simulink model "generic_IsaacV3"  (R2015a)
settings: Solver=ode3  StartTime=0.0  StopTime=inf  FixedStep=0.001  RelTol=1e-3
values from neighbouring files (symbols this model uses):
  coast_domain = 0.1    [LoadVar.m]
  DifferentialFactor = 0.5    [LoadVar.m]
  g = 9.81    [LoadVar.m]
  GearRatio = 10.364    [LoadVar.m]
  Gr = 10.32    [LoadVar.m]
  Lf = 0.78    [LoadVar.m]
  Lr = 0.745    [LoadVar.m]
  M = 265    [LoadVar.m]
  max_coast_Nm = 0    [LoadVar.m]
  MaxSteeringAngle = 24.635    [LoadVar.m]
  mu_max = 1.5    [LoadVar.m]
  ped_max_limiet = 1    [LoadVar.m]
  pedal_position_maxacc = 0.9    [LoadVar.m]
  Reff = 0.2325    [LoadVar.m]
  regen_activation_kph = 15    [LoadVar.m]
  slewbreak_domain = 0.15    [LoadVar.m]
  Sr = 0.6    [LoadVar.m]
  T_max_Nm = 40    [LoadVar.m]
  T_min_Nm = -15    [LoadVar.m]
  TireRadius = 0.4572/2    (= 0.2286)    [LoadVar.m]
  Tmax = 40    [LoadVar.m]
  TrackLength = 1.534    [LoadVar.m]
  TrackWidth = 1.200    (= 1.2)    [LoadVar.m]
libraries: CarMaker4SL x21, simulink x7
(part 3 of 3)

== system generic_IsaacV3/CarMaker/IPG Vehicle/CarAndTrailer/Trailer/CreateBus Vhcl.Wheel.FR ==
  In1 : Inport
  Bus Creator3 : BusCreator  Inputs=14
  Demux3 : Demux  Outputs=14
  Out1 : Outport
  wires:
  Demux3/14 -> Bus Creator3/14  "Vhcl Wheel FR Trq_WhlBearing"
  Demux3/13 -> Bus Creator3/13  "Vhcl Wheel FR Trq_T2W"
  Demux3/12 -> Bus Creator3/12  "Vhcl Wheel FR SideSlip"
  Demux3/11 -> Bus Creator3/11  "Vhcl Wheel FR LongSlip"
  Demux3/10 -> Bus Creator3/10  "Vhcl Wheel FR vBelt"
  Demux3/9 -> Bus Creator3/9  "Vhcl Wheel FR Fz"
  Demux3/8 -> Bus Creator3/8  "Vhcl Wheel FR Fy"
  Demux3/7 -> Bus Creator3/7  "Vhcl Wheel FR Fx"
  Demux3/6 -> Bus Creator3/6  "Vhcl Wheel FR r_zxy z"
  Demux3/5 -> Bus Creator3/5  "Vhcl Wheel FR r_zxy y"
  Demux3/4 -> Bus Creator3/4  "Vhcl Wheel FR r_zxy x"
  Demux3/3 -> Bus Creator3/3  "Vhcl Wheel FR t z"
  Demux3/2 -> Bus Creator3/2  "Vhcl Wheel FR t y"
  In1/1 -> Demux3/1
  Bus Creator3/1 -> Out1/1
  Demux3/1 -> Bus Creator3/1  "Vhcl Wheel FR t x"

== system generic_IsaacV3/CarMaker/IPG Vehicle/CarAndTrailer/Trailer/CreateBus Vhcl.Wheel.RL ==
  In1 : Inport
  Bus Creator3 : BusCreator  Inputs=14
  Demux3 : Demux  Outputs=14
  Out1 : Outport
  wires:
  Demux3/14 -> Bus Creator3/14  "Vhcl Wheel RL Trq_WhlBearing"
  Demux3/13 -> Bus Creator3/13  "Vhcl Wheel RL Trq_T2W"
  Demux3/12 -> Bus Creator3/12  "Vhcl Wheel RL SideSlip"
  Demux3/11 -> Bus Creator3/11  "Vhcl Wheel RL LongSlip"
  Demux3/10 -> Bus Creator3/10  "Vhcl Wheel RL vBelt"
  Demux3/9 -> Bus Creator3/9  "Vhcl Wheel RL Fz"
  Demux3/8 -> Bus Creator3/8  "Vhcl Wheel RL Fy"
  Demux3/7 -> Bus Creator3/7  "Vhcl Wheel RL Fx"
  Demux3/6 -> Bus Creator3/6  "Vhcl Wheel RL r_zxy z"
  Demux3/5 -> Bus Creator3/5  "Vhcl Wheel RL r_zxy y"
  Demux3/4 -> Bus Creator3/4  "Vhcl Wheel RL r_zxy x"
  Demux3/3 -> Bus Creator3/3  "Vhcl Wheel RL t z"
  Demux3/2 -> Bus Creator3/2  "Vhcl Wheel RL t y"
  In1/1 -> Demux3/1
  Bus Creator3/1 -> Out1/1
  Demux3/1 -> Bus Creator3/1  "Vhcl Wheel RL t x"

== system generic_IsaacV3/CarMaker/IPG Vehicle/CarAndTrailer/Trailer/CreateBus Vhcl.Wheel.RR ==
  In1 : Inport
  Bus Creator3 : BusCreator  Inputs=14
  Demux3 : Demux  Outputs=14
  Out1 : Outport
  wires:
  Demux3/14 -> Bus Creator3/14  "Vhcl Wheel RR Trq_WhlBearing"
  Demux3/13 -> Bus Creator3/13  "Vhcl Wheel RR Trq_T2W"
  Demux3/12 -> Bus Creator3/12  "Vhcl Wheel RR SideSlip"
  Demux3/11 -> Bus Creator3/11  "Vhcl Wheel RR LongSlip"
  Demux3/10 -> Bus Creator3/10  "Vhcl Wheel RR vBelt"
  Demux3/9 -> Bus Creator3/9  "Vhcl Wheel RR Fz"
  Demux3/8 -> Bus Creator3/8  "Vhcl Wheel RR Fy"
  Demux3/7 -> Bus Creator3/7  "Vhcl Wheel RR Fx"
  Demux3/6 -> Bus Creator3/6  "Vhcl Wheel RR r_zxy z"
  Demux3/5 -> Bus Creator3/5  "Vhcl Wheel RR r_zxy y"
  Demux3/4 -> Bus Creator3/4  "Vhcl Wheel RR r_zxy x"
  Demux3/3 -> Bus Creator3/3  "Vhcl Wheel RR t z"
  Demux3/2 -> Bus Creator3/2  "Vhcl Wheel RR t y"
  In1/1 -> Demux3/1
  Bus Creator3/1 -> Out1/1
  Demux3/1 -> Bus Creator3/1  "Vhcl Wheel RR t x"

== system generic_IsaacV3/CarMaker/TorqueVectoring/Post-processor/Fysische beperkingen/Lineaire programmering code ==
  Ground{,1..3} (4 alike) : Ground
  Lineaire programering : MATLAB Function  TreatAsAtomicUnit=on
  Terminator : Terminator
  Terminator1 : Terminator
  wires:
  Lineaire programering/2(Trr) -> Terminator1/1
  Lineaire programering/1(Trl) -> Terminator/1
  Ground/1 -> Lineaire programering/1(Trl_maxB)
  Ground2/1 -> Lineaire programering/3(Mz)
  Ground3/1 -> Lineaire programering/4(Tgevraagd)
  Ground1/1 -> Lineaire programering/2(Trr_maxB)

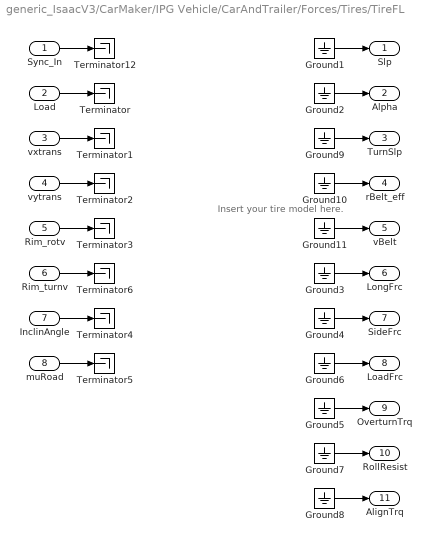
== system generic_IsaacV3/CarMaker/IPG Vehicle/CarAndTrailer/Forces/Tires/TireFL ==
  note: Insert your tire model here.
  Sync_In : Inport
  Load : Inport  Port=2
  vxtrans : Inport  Port=3
  vytrans : Inport  Port=4
  Rim_rotv : Inport  Port=5
  Rim_turnv : Inport  Port=6
  InclinAngle : Inport  Port=7
  muRoad : Inport  Port=8
  Ground{1..11} (11 alike) : Ground
  Terminator{,1..6,12} (8 alike) : Terminator
  Slp : Outport
  Alpha : Outport  Port=2
  TurnSlp : Outport  Port=3
  rBelt_eff : Outport  Port=4
  vBelt : Outport  Port=5
  LongFrc : Outport  Port=6
  SideFrc : Outport  Port=7
  LoadFrc : Outport  Port=8
  OverturnTrq : Outport  Port=9
  RollResist : Outport  Port=10
  AlignTrq : Outport  Port=11
  wires:
  Ground11/1 -> vBelt/1
  Ground10/1 -> rBelt_eff/1
  Ground9/1 -> TurnSlp/1
  Rim_turnv/1 -> Terminator6/1
  Sync_In/1 -> Terminator12/1
  Ground2/1 -> Alpha/1
  Ground3/1 -> LongFrc/1
  Ground4/1 -> SideFrc/1
  Ground5/1 -> OverturnTrq/1
  vxtrans/1 -> Terminator1/1
  vytrans/1 -> Terminator2/1
  Rim_rotv/1 -> Terminator3/1
  InclinAngle/1 -> Terminator4/1
  muRoad/1 -> Terminator5/1
  Load/1 -> Terminator/1
  Ground1/1 -> Slp/1
  Ground6/1 -> LoadFrc/1
  Ground7/1 -> RollResist/1
  Ground8/1 -> AlignTrq/1

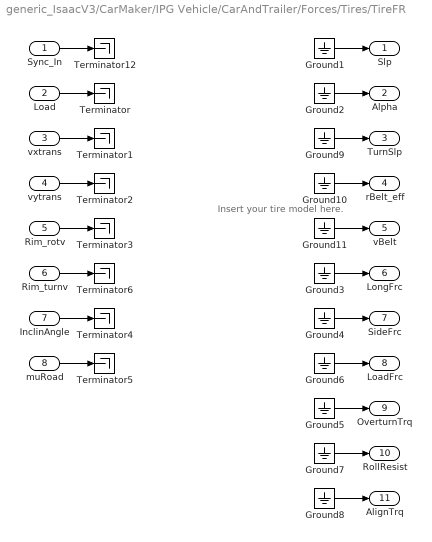
== system generic_IsaacV3/CarMaker/IPG Vehicle/CarAndTrailer/Forces/Tires/TireFR ==
  note: Insert your tire model here.
  Sync_In : Inport
  Load : Inport  Port=2
  vxtrans : Inport  Port=3
  vytrans : Inport  Port=4
  Rim_rotv : Inport  Port=5
  Rim_turnv : Inport  Port=6
  InclinAngle : Inport  Port=7
  muRoad : Inport  Port=8
  Ground{1..11} (11 alike) : Ground
  Terminator{,1..6,12} (8 alike) : Terminator
  Slp : Outport
  Alpha : Outport  Port=2
  TurnSlp : Outport  Port=3
  rBelt_eff : Outport  Port=4
  vBelt : Outport  Port=5
  LongFrc : Outport  Port=6
  SideFrc : Outport  Port=7
  LoadFrc : Outport  Port=8
  OverturnTrq : Outport  Port=9
  RollResist : Outport  Port=10
  AlignTrq : Outport  Port=11
  wires:
  Ground11/1 -> vBelt/1
  Ground10/1 -> rBelt_eff/1
  Ground9/1 -> TurnSlp/1
  Rim_turnv/1 -> Terminator6/1
  Sync_In/1 -> Terminator12/1
  Ground2/1 -> Alpha/1
  Ground3/1 -> LongFrc/1
  Ground4/1 -> SideFrc/1
  Ground5/1 -> OverturnTrq/1
  vxtrans/1 -> Terminator1/1
  vytrans/1 -> Terminator2/1
  Rim_rotv/1 -> Terminator3/1
  InclinAngle/1 -> Terminator4/1
  muRoad/1 -> Terminator5/1
  Load/1 -> Terminator/1
  Ground1/1 -> Slp/1
  Ground6/1 -> LoadFrc/1
  Ground7/1 -> RollResist/1
  Ground8/1 -> AlignTrq/1

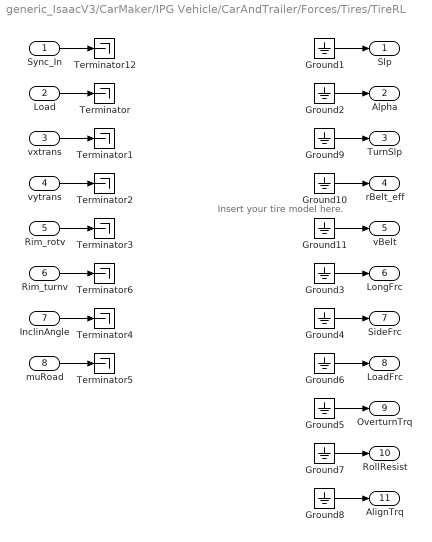
== system generic_IsaacV3/CarMaker/IPG Vehicle/CarAndTrailer/Forces/Tires/TireRL ==
  note: Insert your tire model here.
  Sync_In : Inport
  Load : Inport  Port=2
  vxtrans : Inport  Port=3
  vytrans : Inport  Port=4
  Rim_rotv : Inport  Port=5
  Rim_turnv : Inport  Port=6
  InclinAngle : Inport  Port=7
  muRoad : Inport  Port=8
  Ground{1..11} (11 alike) : Ground
  Terminator{,1..6,12} (8 alike) : Terminator
  Slp : Outport
  Alpha : Outport  Port=2
  TurnSlp : Outport  Port=3
  rBelt_eff : Outport  Port=4
  vBelt : Outport  Port=5
  LongFrc : Outport  Port=6
  SideFrc : Outport  Port=7
  LoadFrc : Outport  Port=8
  OverturnTrq : Outport  Port=9
  RollResist : Outport  Port=10
  AlignTrq : Outport  Port=11
  wires:
  Ground11/1 -> vBelt/1
  Ground10/1 -> rBelt_eff/1
  Ground9/1 -> TurnSlp/1
  Rim_turnv/1 -> Terminator6/1
  Sync_In/1 -> Terminator12/1
  Ground2/1 -> Alpha/1
  Ground3/1 -> LongFrc/1
  Ground4/1 -> SideFrc/1
  Ground5/1 -> OverturnTrq/1
  vxtrans/1 -> Terminator1/1
  vytrans/1 -> Terminator2/1
  Rim_rotv/1 -> Terminator3/1
  InclinAngle/1 -> Terminator4/1
  muRoad/1 -> Terminator5/1
  Load/1 -> Terminator/1
  Ground1/1 -> Slp/1
  Ground6/1 -> LoadFrc/1
  Ground7/1 -> RollResist/1
  Ground8/1 -> AlignTrq/1

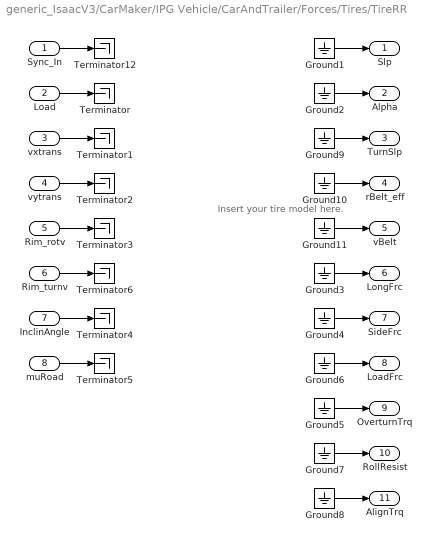
== system generic_IsaacV3/CarMaker/IPG Vehicle/CarAndTrailer/Forces/Tires/TireRR ==
  note: Insert your tire model here.
  Sync_In : Inport
  Load : Inport  Port=2
  vxtrans : Inport  Port=3
  vytrans : Inport  Port=4
  Rim_rotv : Inport  Port=5
  Rim_turnv : Inport  Port=6
  InclinAngle : Inport  Port=7
  muRoad : Inport  Port=8
  Ground{1..11} (11 alike) : Ground
  Terminator{,1..6,12} (8 alike) : Terminator
  Slp : Outport
  Alpha : Outport  Port=2
  TurnSlp : Outport  Port=3
  rBelt_eff : Outport  Port=4
  vBelt : Outport  Port=5
  LongFrc : Outport  Port=6
  SideFrc : Outport  Port=7
  LoadFrc : Outport  Port=8
  OverturnTrq : Outport  Port=9
  RollResist : Outport  Port=10
  AlignTrq : Outport  Port=11
  wires:
  Ground11/1 -> vBelt/1
  Ground10/1 -> rBelt_eff/1
  Ground9/1 -> TurnSlp/1
  Rim_turnv/1 -> Terminator6/1
  Sync_In/1 -> Terminator12/1
  Ground2/1 -> Alpha/1
  Ground3/1 -> LongFrc/1
  Ground4/1 -> SideFrc/1
  Ground5/1 -> OverturnTrq/1
  vxtrans/1 -> Terminator1/1
  vytrans/1 -> Terminator2/1
  Rim_rotv/1 -> Terminator3/1
  InclinAngle/1 -> Terminator4/1
  muRoad/1 -> Terminator5/1
  Load/1 -> Terminator/1
  Ground1/1 -> Slp/1
  Ground6/1 -> LoadFrc/1
  Ground7/1 -> RollResist/1
  Ground8/1 -> AlignTrq/1

== stateflow chart generic_IsaacV3/CarMaker/PedalMapping/Chart ==
  state LaunchSet
    entry:
    pedal=0;
    during:
    pedal=0;
    DRS_S2=0;
    DRS_S3=0;
  state LaunchGo
    during:
    pedal=ped_pos;
    DRS_S2=0;
    DRS_S3=0;
  (default) -> LaunchSet
  LaunchSet -> LaunchGo : [LC==1 && ped_pos>=0.8]
  LaunchGo -> LaunchSet : [LC==0]
  data: ped_pos input; pedal output; DRS_S2 output; DRS_S3 output; LC input

== stateflow chart generic_IsaacV3/CarMaker/Traction Control Logic ==
  state Launch
    entry:
    T_OutRR_Nm=0;
    T_OutRL_Nm=0;
    during:
    T_OutRL_Nm=Tin_ped;
    T_OutRR_Nm=Tin_ped;
  state Torque_Vectoring
    during:
    T_OutRL_Nm=Tin_TV_RL;
    T_OutRR_Nm=Tin_TV_RR;
  state Launch_Control
    entry:
    T_OutRL_Nm=0;
    T_OutRR_Nm=0;
    during:
    T_OutRL_Nm=Tin_SC_RL;
    T_OutRR_Nm=Tin_SC_RR;
  state Slip_Control
    during:
    T_OutRL_Nm=Tin_SC_RL;
    T_OutRR_Nm=Tin_SC_RR;
  (default) -> Launch
  Launch -> Launch_Control [order 2] : [LC==1]
  Launch_Control -> Launch : [LC==0]
  Launch -> Slip_Control [order 3] : [SC==1]
  Torque_Vectoring -> Launch [order 2] : [TV==0]
  Launch -> Torque_Vectoring [order 1] : [TV==1]
  Slip_Control -> Torque_Vectoring [order 1] : [Steering_Angle>10 && TV==1||SC==0]
  Torque_Vectoring -> Slip_Control [order 1] : [Steering_Angle<10 && SC==1]
  Slip_Control -> Launch_Control [order 2] : [LC==1]
  data: T_OutRL_Nm output; Tin_ped input; T_OutRR_Nm output; Steering_Angle input; SC input; TV input; LC input; Tin_TV_RL input; Tin_TV_RR input; Tin_SC_RL input; Tin_SC_RR input

== matlab function generic_IsaacV3/CarMaker/SignalOut/MATLAB Function ==
  data: Wheelspeed_Max input; T_mot output; Wheelspeed_Sens input; Treq input
function T_mot = SpeedLimit(Wheelspeed_Max,Wheelspeed_Sens,Treq)
%Speed limiter for IPG Carmaker
if Wheelspeed_Sens>= Wheelspeed_Max
    T_mot=0;
else
    T_mot=Treq;
end

== matlab function generic_IsaacV3/CarMaker/PedalMapping/vehicle velocity fun ==
  data: wheelspeedfl input; v_vehicle_mps output; wheelspeedfr input; v_vehicle_kph output
function [v_vehicle_mps,v_vehicle_kph] = vehicle_velocity(wheelspeedfl,wheelspeedfr)
%% vehicle speed estimation
r=0.2286;

v_vehicle_mps= (wheelspeedfl+wheelspeedfr)/2 *r;
v_vehicle_kph=v_vehicle_mps*3.6;

== matlab function generic_IsaacV3/CarMaker/SignalOut/MATLAB Function1 ==
  data: Wheelspeed_Max input; T_mot output; Wheelspeed_Sens input; Treq input
function T_mot = SpeedLimit(Wheelspeed_Max,Wheelspeed_Sens,Treq)
%Speed limiter for IPG Carmaker
if Wheelspeed_Sens>= Wheelspeed_Max
    T_mot=0;
else
    T_mot=Treq;
end

== matlab function generic_IsaacV3/CarMaker/MTTE Slipcontrol/Max wheel torque estimator1 ==
  data: Fd input; Twheel output; w_FL input; w_FR input; SR input; a_chassis input; v_chassis output
function [Twheel,v_chassis] = TorqueEstimation(Fd,w_FL,w_FR,SR,a_chassis)
%% estimator wheel torque

Jw =0.0275; %[kgm²] Massatraagheid wiel (roterende componenten)
r=0.2286; %[m] straal wiel
a=0.9; %relacation factor a=Vchasis/Vwheel

Tmax= 400; %[Nm] Wheel Torque

w_chassis=(w_FL+w_FR)/2; % average speed
v_chassis=w_chassis*r; %[m/s] velocity of the chasis

if SR <0.05
    Twheel=Tmax;
else
    Twheel = max(a_chassis*Jw/(a*r)+r*Fd,100);
end

== matlab function generic_IsaacV3/CarMaker/MTTE Slipcontrol/Max wheel torque estimator ==
  data: Fd input; Twheel output; w_FL input; w_FR input; SR input; a_chassis input; v_chassis output
function [Twheel,v_chassis] = TorqueEstimation(Fd,w_FL,w_FR,SR,a_chassis)
%% estimator wheel torque

Jw =0.0275; %[kgm²] Massatraagheid wiel (roterende componenten)
r=0.2286; %[m] straal wiel
a=0.9; %relacation factor a=Vchasis/Vwheel

Tmax= 400; %[Nm] Wheel Torque

w_chassis=(w_FL+w_FR)/2; % average speed
v_chassis=w_chassis*r; %[m/s] velocity of the chasis

if SR <0.05
    Twheel=Tmax;
else
    Twheel = max(a_chassis*Jw/(a*r)+r*Fd,100);
end

== matlab function generic_IsaacV3/CarMaker/Vehicle Sensors/PreProcessor/MATLAB Function ==
  data: speedfl input; slip_ratio_gem output; speedfr input; speedrl input; speedrr input; vehicle_speed_mps output; slip_ratio_RL output; slip_ratio_RR output
function [slip_ratio_gem, vehicle_speed_mps,slip_ratio_RL,slip_ratio_RR]=Launch_slip_calc(speedfl,speedfr,speedrl,speedrr)
%Calculates the wheel slip ratio

rwheel=0.2286; %m
e = 0.01; %Low speed smoothing

Rotspeed_front=(speedfl+speedfr)/2; %[rad/s]average rotational speed front
Rotspeed_rear = max(speedrl,speedrr);%[rad/s]average rotational speed rear

vehicle_speed_mps=Rotspeed_front*rwheel; %[m/s] vehicle speed

slip_ratio_gem=(1-vehicle_speed_mps/(rwheel*Rotspeed_rear));

slip_ratio_RL=(rwheel*speedrl-vehicle_speed_mps)/max((rwheel*speedrl),e);
slip_ratio_RR=(rwheel*speedrr-vehicle_speed_mps)/max((rwheel*speedrr),e);

if slip_ratio_gem<0
    slip_ratio_gem=0;
end

end

== matlab function generic_IsaacV3/CarMaker/E-diff/ThrottleStatus ==
  data: CurrentTorqueRequest input; ArrayPrevious input; Accelerating output; ArrayNext output
function [Accelerating, ArrayNext] = MovingAverage(CurrentTorqueRequest, ArrayPrevious)
% Calculates the moving average of the matrix defined in the memory block

% Calculation of moving average
TorqueAverage = mean(ArrayPrevious);
ArrayNext = circshift(ArrayPrevious,1);
ArrayNext(1) = CurrentTorqueRequest;

% Looks whether the current torque request exceeds the mean of the previous 100ms torque commands
if CurrentTorqueRequest > TorqueAverage && CurrentTorqueRequest > 0
    Accelerating = 1;
else
    Accelerating = 0;
end

== matlab function generic_IsaacV3/CarMaker/TorqueVectoring/Post-processor/Fysische beperkingen/Lineaire programmering code/Lineaire programering ==
  data: Trl_maxB input; Trl output; Trr_maxB input; Mz input; Tgevraagd input; Trr output
function [Trl,Trr] = Lineaire_programmering(Trl_maxB,Trr_maxB,Mz,Tgevraagd)
%Dit blok staat in voor het berekenen van het te leveren koppel per wiel
%aan de hand van twee lineaire doelen. Het eerste doel is het gewenst 
%koppel om rechtdoor te rijden. Het tweede doel is het berekende moment van 
%de PI-regelaar om te zetten naar een koppelverschil van maximaal 10 Nm 
%over de twee achterwielen.
%Als de twee doelen berekend zijn worden ze opgeteld om tot het
%resulterende koppel per wiel te komen. Deze koppels worden naar het
%wagenmodel of de motordrives van de effectieve wagen gestuurd.

%%
%Parameters
Reff	=0.2325;            
Gr      =10.32;             
Sr      =0.600;                 

%%
%Eerste versie

%Gevraagd koppel rechtdoor
Trl_maxM = Trl_maxB/Gr;
Trr_maxM = Trr_maxB/Gr;

Trl_1 = min(Trl_maxM,Tgevraagd);
Trr_1 = min(Trr_maxM,Tgevraagd);

%Gevraagd moment om z-as
T_delta = (Mz*Reff)/(2*Sr*Gr) ;

Trl_2 = T_delta;
Trr_2 = -T_delta;

%Totaal koppel
Trl = Trl_1 + Trl_2;
Trr = Trr_1 + Trr_2;

== matlab function generic_IsaacV3/CarMaker/TorqueVectoring/Post-processor/Slip-controle  ==
  data: ax input; ay input; mu_max input; A output; Vzwp input; B output; C output; D output; Wf output; Wr output
function [A,B,C,D,Wf,Wr] = Slip_controle(ax,ay,mu_max,Vzwp)
% Berekening van de maximale torques die men kan toepassen op de wielen
% door berekening van de normaalkrachten op de wielen.

%load('parameters.mat');

M       = 265;             
L       = 1.525;                           
Lf      = 0.780;                              
Lr      = 0.745;                              
Tf      = 1.200;                             
Tr      = 1.200;                            
g       = 9.81;                                                       
Krf_a	= 183.26;                            
Krr_a	= 325.31;                           
Ksf     = 12153;             %Veerstijfheid vooraan
Ksr     = 14563;
H       = 0.2735;                        
    %ax      =0;                 
    %ay      =0;                               
    %Vzwp    =0;                 
    %mu_max  =1.5;

%Wielbelastingen

%Statische wielbelasting
Ws_fl = ((Lr*M*g)/(2*L));
Ws_fr = ((Lr*M*g)/(2*L));
Ws_rl = ((Lf*M*g)/(2*L));
Ws_rr = ((Lf*M*g)/(2*L));

%Ws_f = Ws_fl + Ws_fr;
%Ws_r = Ws_rl + Ws_rr;

%Laterale wielbelasting (door rollen van de wagen)
Wy_fl = -((H*M*ay)/(2*Tf));                         %Kracht per wiel
Wy_fr =  ((H*M*ay)/(2*Tf));
Wy_rl = -((H*M*ay)/(2*Tr));
Wy_rr =  ((H*M*ay)/(2*Tr));

%Longitudinale wielbelasting
Wx_fl = -((H*M*ax)/(2*L));                          %Kracht per wiel
Wx_fr = -((H*M*ax)/(2*L));
Wx_rl =  ((H*M*ax)/(2*L));
Wx_rr =  ((H*M*ax)/(2*L));

%Aerodynamische wielbelasting
LF = -0.0237*(Vzwp)^2 + 0.0958*Vzwp;                %Nog na te kijken; komt uit excel van aeromannen
LR = -0.0237*(Vzwp)^2 + 0.0958*Vzwp;                %Nog na te kijken; komt uit excel van aeromannen

Wa_fl = (-LF/2);  %+((Krf/(Krf+Krr))*(Rm/Tf));      %is er hier 2x rolmoment??? (zie lateraal)
Wa_fr = (-LF/2);  %-((Krf/(Krf+Krr))*(Rm/Tf));
Wa_rl = (-LR/2);  %+((Krr/(Krf+Krr))*(Rm/Tr));
Wa_rr = (-LR/2);  %-((Krr/(Krf+Krr))*(Rm/Tr));

%anti-roll bar wielbelasting
Wab_fl =  ((Krf_a*(-Wy_fl))/((Krf_a+((Ksf*(Tf)^2)/2))));
Wab_fr =  ((Krf_a*(-Wy_fr))/((Krf_a+((Ksf*(Tf)^2)/2))));
Wab_rl =  ((Krr_a*(-Wy_rl))/((Krr_a+((Ksr*(Tr)^2)/2))));
Wab_rr =  ((Krr_a*(-Wy_rr))/((Krr_a+((Ksr*(Tr)^2)/2))));

%Totale belasting per wiel
Wfl = Ws_fl + Wy_fl + Wx_fl + Wa_fl + Wab_fl;   %Ongebruikt, kan later eventueel gebruikt worden voor 4WD??
Wfr = Ws_fr + Wy_fr + Wx_fr + Wa_fr + Wab_fr;   %^ Idem
Wrl = Ws_rl + Wy_rl + Wx_rl + Wa_rl + Wab_rl;
Wrr = Ws_rr + Wy_rr + Wx_rr + Wa_rr + Wab_rr;



%%Omrekening naar torques
%HIER GEWIJZIGD

%Wrijvingscirkels (wortels worden naar buiten gebracht; kunnen niet
%berekend worden in code; geeft fouten; vervolgens ook vermenigvuldigen 
%met effectieve bandenstraal om tot de wielkoppels te komen)

%Jx_rl = ((Wrl*mu_max)^2-((Wrl*ay)/(g))^2);
%Jx_rr = ((Wrr*mu_max)^2-((Wrr*ay)/(g))^2);

%     if Jx_rl < 0
%     then Jx_rl = 0
% end
% 
% if Jx_rr < 0
%     then Jx_rr = 0
% end


A = (Wrl*mu_max)^2;
B = ((Wrl*ay)/(g))^2;
C = (Wrr*mu_max)^2;
D = ((Wrr*ay)/(g))^2;

% Fx_rl = sqrt((Wrl*mu_max)^2-((Wrl*ay)/(g))^2);
% 
% Fx_rr = sqrt((Wrr*mu_max)^2-((Wrr*ay)/(g))^2);

%Maximum torques
% Trl_max = Fx_rl*Reff;
% Trr_max = Fx_rr*Reff;

%Belastingen per as
Wf = (Wfl+Wfr)/2;
Wr = (Wrl+Wrr)/2;

== matlab function generic_IsaacV3/CarMaker/TorqueVectoring/Pre-processor/prepros - code/Pre-processor ==
  data: Yaw_ref output; Vzwp input; stuurhoek input; mu_max input; a_zwpx input; Fy_f input; Fy_r input; alfa_r1 input; alfa_f output; alfa_r output; alfa_f1 input
function [Yaw_ref,alfa_f,alfa_r]= pre_processor(Vzwp,stuurhoek,mu_max,a_zwpx,Fy_f,Fy_r,alfa_r1,alfa_f1)
%De pre-processor berekend de gewenste yaw rate door het minimum te nemen
%van de ideale en de maximale yaw rate waarde.
%Belangrijk hierbij de hoeken in RAD!!!!!!

%Parameters
M       = 265;             
L       = 1.525;                           
Lf      = 0.780;                              
Lr      = 0.745; 
g       = 9.81;

%Berekening massa's
Wf = (M*Lr*g/L);
Wr = (M*Lf*g/L);

% berekening van de sliphoek beita
beita = atan(Lf * tan(stuurhoek)/ (Lf+Lr)) ;



%Berekening Cornering stiffness
               Cf = (Fy_f/alfa_f1);
               Cr = (Fy_r/alfa_r1);
%              C_rl = (Fy_rl/alfa_rl);
%              C_rr = (Fy_rr/alfa_rr);
                
 % Fy_f = Cf * alfa_f ;
 % Fy_r = Cr * alfa_r ;
%Gemiddelde van de cornering stiffness vooraan en achteraan nemen
          %Cf = ((C_fl + C_fr)/ 2);
          %Cr = ((C_rl + C_rr)/ 2);
%Berekening van de onderstuur factor.
Ku = ((Wf/Cf)-(Wr/Cr));

%Berekening van de ideale yaw rate.
Yaw_id = ((Vzwp*stuurhoek)/((Lf+Lr)+Ku*(Vzwp)^2));

%Berekening van de maximale yaw rate.
Yaw_max = (((mu_max*g)-(a_zwpx * tan(beita)) - (Vzwp * cos(beita)* diff(beita)))/(Vzwp*cos(beita)));

%Minimale yaw rate.
Yaw_ref = min([Yaw_id ; Yaw_max]);
%Berekening sliphoeken
alfa_f = - beita + stuurhoek - ((Lf * Yaw_ref)/Vzwp);
alfa_r = - beita + ((Lr * Yaw_ref)/Vzwp);

== stateflow chart generic_IsaacV3/CarMaker/E-diff/Differential_Statemachine ==
  state Offline
    entry:
    DMC1_SpeedRq = 14000;
    DMC2_SpeedRq = 14000;
  state Standby
    entry:
    DMC1_SpeedRq = 14000;
    DMC2_SpeedRq = 14000;
  state Online
    entry:
    DMC1_SpeedRq = SpeedRq1;
    DMC2_SpeedRq = SpeedRq2;
  (default) -> Offline
  (junction 28) -> Offline : [EnableDifferential == 0 || SteeringAngleError == 1 || WheelSpeedError == 1]
  Offline -> Standby : [EnableDifferential == 1 && SteeringAngleError == 0 && WheelSpeedError == 0]
  Standby -> (junction 28) [order 2]
  Online -> (junction 28) [order 2]
  Online -> Standby [order 1] : [abs(SteeringAngle) < 3]
  Standby -> Online [order 1] : [abs(SteeringAngle) > 2]
  data: EnableDifferential input; SteeringAngle input; WheelSpeedError input; SteeringAngleError input; SpeedRq1 input; SpeedRq2 input; DMC1_SpeedRq output; DMC2_SpeedRq output

== matlab function generic_IsaacV3/CarMaker/E-diff/E-Differential/Differential ==
  data: Accelerating input; MaxSpeedRight_rpm output; MaxSpeedLeft_rpm output; SteeringAngle input; Velocity input; DifferentialFactor input; MaxSteeringAngle input; TrackWidth input; TrackLength input; GearRatio input; TireRadius input
function [MaxSpeedRight_rpm,MaxSpeedLeft_rpm] = Differential(Accelerating,SteeringAngle, Velocity, DifferentialFactor,MaxSteeringAngle,TrackWidth,TrackLength,GearRatio,TireRadius)
% Positive Turn = Right Turn
% Negative Turn = Left Turn

TurnRadius =  TrackLength/tan(SteeringAngle*pi/180); % R in m
if Accelerating == 1
    TurnSpeed = (Velocity + DifferentialFactor*(MaxSteeringAngle-abs(SteeringAngle))/MaxSteeringAngle)/TurnRadius; % Omega in rad/s
else
    TurnSpeed = Velocity/TurnRadius; % Omega in rad/s
end

MaxSpeedRight_mps = (TurnRadius - TrackWidth/2)*TurnSpeed; % V_r in m/s
MaxSpeedLeft_mps = (TurnRadius + TrackWidth/2)*TurnSpeed; % V_l in m/s        

MaxSpeedRight_rpm = MaxSpeedRight_mps/TireRadius*60/2/pi*GearRatio; % V_r in rpm
MaxSpeedLeft_rpm = MaxSpeedLeft_mps/TireRadius*60/2/pi*GearRatio; % V_l in rpm

== matlab function generic_IsaacV3/CarMaker/E-diff/VelocityStatus ==
  data: CurrentVelocity input; ArrayPrevious input; Accelerating output; ArrayNext output
function [Accelerating, ArrayNext] = MovingAverage(CurrentVelocity, ArrayPrevious)
% Calculates the moving average of the matrix defined in the memory block

% Calculation of moving average
VelocityAverage = mean(ArrayPrevious);
ArrayNext = circshift(ArrayPrevious,1);
ArrayNext(1) = CurrentVelocity;

% Looks whether the current torque request exceeds the mean of the previous 100ms torque commands
if CurrentVelocity > VelocityAverage && CurrentVelocity > 0
    Accelerating = 1;
else
    Accelerating = 0;
end

== matlab function generic_IsaacV3/CarMaker/PedalMapping/Pedal map1 ==
  data: ped_pos input; coast_dom input; T_out output; slewbreak_dom input; ped_accel input; ped_max input; ped_max_limit input; T_max input; T_min input; T_coast input
function T_out = Pedalmap_eq(ped_pos,coast_dom,slewbreak_dom,ped_accel,ped_max,ped_max_limit,T_max,T_min,T_coast)
%%Accelerator pedal mapping:

ped_regen=ped_accel-coast_dom; %pedal postion - start regen - variable in function of velocity
ped_zero=ped_regen-slewbreak_dom; %pedal postion - start max regen - variable in function of velocity

slewrate_acc=(T_max-T_coast)/(ped_max-ped_accel); %slewrate acceleration region
slewrate_regen=(T_min-T_coast)/(ped_zero-ped_regen);%slewrate regen region

% acceleration pedal map eq.
T_out=T_min*(heavi(ped_pos,-0.1)-heavi(ped_pos,ped_zero)) + (slewrate_regen*(ped_pos-ped_regen)+T_coast)*(heavi(ped_pos,ped_zero)-heavi(ped_pos,ped_regen))+T_coast*(heavi(ped_pos,ped_regen)-heavi(ped_pos,ped_accel))+(slewrate_acc*(ped_pos-ped_accel)+T_coast)*(heavi(ped_pos,ped_accel)-heavi(ped_pos,ped_max))+T_max*(heavi(ped_pos,ped_max-heavi(ped_pos,ped_max_limit)));

== stateflow chart generic_IsaacV3/CarMaker/PedalMapping/pedal logic1 ==
  state Driving
    state Disable_regen
      entry:
      ped_accel=0.45;
      T_regen=0;
    state Activate_regen
      entry:
      ped_accel=0.45;
      T0= -5; %Regentorque at v_lim [Nm]
      during:
      % velocity dependant braking torque
      if v_vehicle<15
      T_regen=T_min/(15-5)*(v_vehicle-5);
      elseif v_vehicle<50
      T_regen=T_min;
      else
      T_regen=min((T_min-T0)/(50-100)*(v_vehicle-100)+T0,0);
      end
    (default) -> Disable_regen
    Disable_regen -> Activate_regen : [SoC<0.95 && Enable_regen==1]
    Activate_regen -> Disable_regen : [SoC>0.95 || T_cell>55 || Enable_regen==0]
  state Standstill
    entry:
    T_regen=0;
    ped_accel=0.1; %
    during:
    %velocity dependent coasting until v_max
    ped_accel=min(max(ped_pos* (v_vehicle/v_max),0.1),0.45); %Offset of 0.1
    exit:
    ped_accel=0.45;
  (default) -> Standstill
  Driving -> Standstill : [v_vehicle<=5]
  Standstill -> Driving : [v_vehicle >v_max&&ped_pos>0.45]
  data: T_min input; SoC input; v_max input; ped_pos input; v_vehicle input; ped_accel output; T_regen output; T0 local; T_cell input; Enable_regen input
